simulink library "g_block"  (R2024b)
settings: Solver=VariableStepAuto  StartTime=0.0  StopTime=10.0  RelTol=1e-3
settings Model: Creator=pinto  LastModifiedBy=pinto

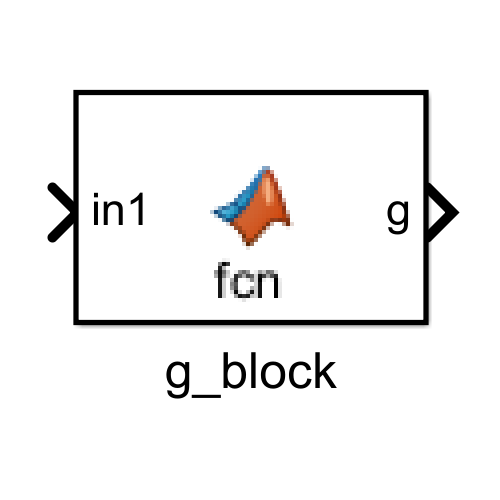
[thumbnail: Simulink's stored preview of the top-level diagram]
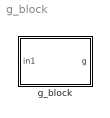
== system g_block ==
  g_block : MATLAB Function  TreatAsAtomicUnit=on

== matlab function g_block/g_block ==
  data: in1 input; g output
function g = g_block(in1)
%#codegen

%    This function was generated by the Symbolic Math Toolbox version 24.2.
%    17-Jun-2025 19:47:26

% in1 = complex(in1);  % if required to enforce complex operations
q2 = in1(2,:);
q3 = in1(3,:);
q4 = in1(4,:);
t2 = cos(q2);
t3 = cos(q4);
t4 = sin(q2);
t5 = sin(q3);
t6 = sin(q4);
g = [0.0;t2.*1.881760140925538e+1+t2.*t3.*3.390811274043039+t4.*t5.*t6.*3.390811274043039;t2.*t6.*cos(q3).*(-3.390811274043039);t4.*t6.*(-3.390811274043039)-t2.*t3.*t5.*3.390811274043039;0.0];
end
